simulink model "CruiseCtrl_StateFeedback_Int"  (R2020a)
settings: Solver=ode45  StartTime=0.0  StopTime=40  MaxStep=0.01  RelTol=1e-3  EnableMultiTasking=on
values from neighbouring files (symbols this model uses):
  r = 57    [Driveline_ctrl_design.m]
undefined symbols (not defined in the file or in its folder): Af, CD, f, g, k, Kaug, m, rho, rw, tau, ue, x1e, x2e
settings Model: Creator=JonasMac  LastModifiedBy=juan
settings DataIOCC: LimitDataPoints=on  SaveFormat=Array  ReturnWorkspaceOutputs=off
settings OptimizationCC: LifeSpan=inf
settings DebuggingCC: UnderspecifiedInitializationDetection=Classic  MergeDetectMultiDrivingBlocksExec=none  SolverPrmCheckMsg=warning  SFUnexpectedBacktrackingDiag=warning  SFNoUnconditionalDefaultTransitionDiag=warning  SFExecutionAtInitializationDiag=none  ArithmeticOperatorsInVariantConditions=warning
settings HardwareCC: ProdBitPerPointer=32  ProdBitPerSizeT=32  ProdBitPerPtrDiffT=32  ProdLargestAtomicFloat=None  ProdIntDivRoundTo=Undefined  ProdEndianess=Unspecified  ProdWordSize=32  ProdHWDeviceType=32-bit Generic
settings ModelReferenceCC: PropagateSignalLabelsOutOfModel=off
settings SFSimCC: SimUseLocalCustomCode=off  CustomCodeUndefinedFunction=UseInterfaceOnly
settings RTWCC: RTWUseLocalCustomCode=off
settings CodeAppCC: StateflowObjectComments=on
settings GRTTargetCC: TargetLangStandard=C89/C90 (ANSI)
settings ConfigComp: CovMetricSettings=dw  CovHtmlReporting=on  CovSaveCumulativeToWorkspaceVar=on  CovSaveSingleToWorkspaceVar=on  CovExternalEMLEnable=off

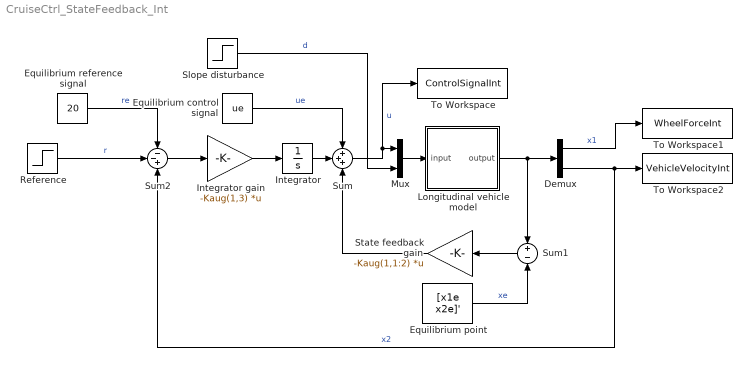
== system CruiseCtrl_StateFeedback_Int ==
  Demux : Demux  Outputs=2
  Equilibrium control signal : Constant  Value=ue
  "Equilibrium point " : Constant  Value=[x1e x2e]'
  Equilibrium reference signal : Constant  Value=20
  Integrator : Integrator
  Integrator gain : Gain  Gain=-Kaug(1,3)  Multiplication=Matrix(K*u)
  Longitudinal vehicle model : Subsystem
  Mux : Mux  Inputs=2
  Reference : Step  After=5  SampleTime=0
  Slope disturbance : Step  Time=20  After=0.1  SampleTime=0
  State feedback gain : Gain  Gain=-Kaug(1,1:2)  Multiplication=Matrix(K*u)
  Sum : Sum  Inputs=+++
  Sum1 : Sum  Inputs=+-
  Sum2 : Sum  Inputs=--+
  To Workspace : ToWorkspace  VariableName=ControlSignalInt  SaveFormat=Structure With Time  SampleTime=-1
  To Workspace1 : ToWorkspace  VariableName=WheelForceInt  SaveFormat=Structure With Time  SampleTime=-1
  To Workspace2 : ToWorkspace  VariableName=VehicleVelocityInt  SaveFormat=Structure With Time  SampleTime=-1
  wires:
  Demux/2 -> Sum2/3, To Workspace2/1  "x2"
  Sum/1 -> To Workspace/1, Mux/1  "u"
  Slope disturbance/1 -> Mux/2  "d"
  Integrator/1 -> Sum/2
  Equilibrium control signal/1 -> Sum/1  "ue"
  Longitudinal vehicle model/1(output) -> Sum1/1, Demux/1
  Mux/1 -> Longitudinal vehicle model/1(input)
  State feedback gain/1 -> Sum/3
  Sum1/1 -> State feedback gain/1
  "Equilibrium point "/1 -> Sum1/2  "xe"
  Sum2/1 -> Integrator gain/1
  Integrator gain/1 -> Integrator/1
  Reference/1 -> Sum2/2  "r"
  Equilibrium reference signal/1 -> Sum2/1  "re"
  Demux/1 -> To Workspace1/1  "x1"

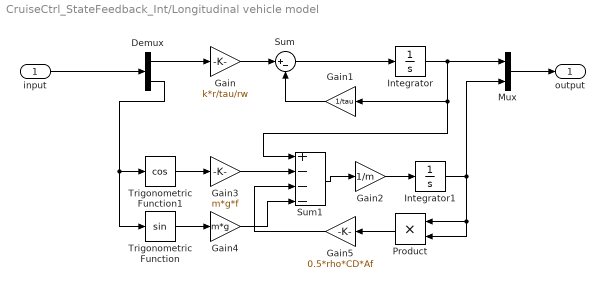
== system CruiseCtrl_StateFeedback_Int/Longitudinal vehicle model ==
  input : Inport
  Demux : Demux  Outputs=2
  Gain : Gain  Gain=k*r/tau/rw
  Gain1 : Gain  Gain=1/tau
  Gain2 : Gain  Gain=1/m
  Gain3 : Gain  Gain=m*g*f
  Gain4 : Gain  Gain=m*g
  Gain5 : Gain  Gain=0.5*rho*CD*Af
  Integrator : Integrator  InitialCondition=x1e
  Integrator1 : Integrator  InitialCondition=x2e
  Mux : Mux  Inputs=2
  Product : Product
  Sum : Sum  Inputs=|+-
  Sum1 : Sum  Inputs=+---
  Trigonometric Function : Trigonometry
  Trigonometric Function1 : Trigonometry  Operator=cos
  output : Outport  VectorParamsAs1DForOutWhenUnconnected=off
  wires:
  Mux/1 -> output/1
  input/1 -> Demux/1
  Integrator/1 -> Sum1/1, Gain1/1, Mux/1
  Integrator1/1 -> Product/2, Product/1, Mux/2
  Demux/1 -> Gain/1
  Gain/1 -> Sum/1
  Sum/1 -> Integrator/1
  Gain1/1 -> Sum/2
  Gain2/1 -> Integrator1/1
  Sum1/1 -> Gain2/1
  Demux/2 -> Trigonometric Function1/1, Trigonometric Function/1
  Trigonometric Function1/1 -> Gain3/1
  Gain3/1 -> Sum1/2
  Trigonometric Function/1 -> Gain4/1
  Gain4/1 -> Sum1/4
  Product/1 -> Gain5/1
  Gain5/1 -> Sum1/3
